simulink model "Detumble_HIL"  (R2020a)
settings: Solver=ode4  StartTime=0.0  StopTime=10  FixedStep=0.05  RelTol=1e-3
values from neighbouring files (symbols this model uses):
  E_b_ECI = [phi_b_ECI; theta_b_ECI; psi_b_ECI]    [Detumble_Initial.m]
  epsilon_b_ECI = [(C_b_ECI(2,3)-C_b_ECI(3,2))/(4*eta_b_ECI) ... (first row only)    [Detumble_Initial.m]
  eta_b_ECI = ((trace(C_b_ECI) + 1)^0.5)/2    [Detumble_Initial.m]
  omega_b_ECI = [-0.05; 0.03; 0.2]    [Detumble_Initial.m]
  state0 = [omega_b_ECI; E_b_ECI; epsilon_b_ECI; eta_b_ECI]    [Detumble_Initial.m]
undefined symbols (not defined in the file or in its folder): Com2, DiscIntNeverNeededParam, none
libraries: xpcseriallib x5
settings Model: SimulationMode=external  Creator=sheab  LastModifiedBy=sheab
settings SolverCC: ConcurrentTasks=on  AutoInsertRateTranBlk=on
settings DataIOCC: SaveFormat=StructureWithTime  SaveOutput=off
settings OptimizationCC: BlockReduction=off  OptimizeBlockIOStorage=off
settings HardwareCC: ProdBitPerPointer=32  ProdBitPerSizeT=32  ProdBitPerPtrDiffT=32  ProdLargestAtomicFloat=None  ProdWordSize=32  ProdLongLongMode=on  ProdHWDeviceType=Generic->32-bit x86 compatible
settings RTWCC: Description=Simulink Real-Time  SystemTargetFile=slrt.tlc  TemplateMakefile=slrt_default_tmf  CodeExecutionProfiling=on  RTWCompilerOptimization=on
settings SimulinkRealTimeCC: SupportVariableSizeSignals=on  RL32LogTETModifier=off  xPCConcurrentTasks=on

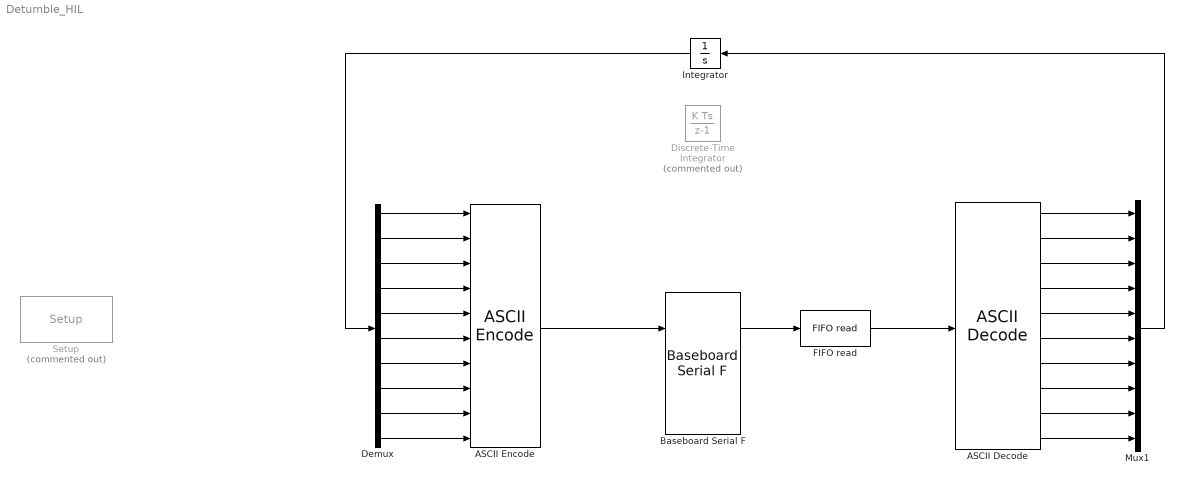
== system Detumble_HIL ==
  "ASCII Decode " : xpcseriallib/ASCII Decode   format=%f %f %f %f %f %f %f %f %f %f\n  nvars=10  vartypes={}
      settings: SourceProductBaseCode=XP
  "ASCII Encode " : xpcseriallib/ASCII Encode   format=%f %f %f %f %f %f %f %f %f %f \n  nvars=10  maxlength=128  vartypes={ 'double' }
      settings: SourceProductBaseCode=XP
  Baseboard Serial F : xpcseriallib/Mainboard/Baseboard Serial F  group=FIFO Setup  port=1  irqnum=4  saddr1=0x3f8  saddr2=0x3e8  config=Com2/none  baud1=115200  parity1=None  ndata1=8  nstop1=1  fifomode1=16 deep  rlevel1=half full  automode1=off  xmtfifosize1=1024  xmtdatatype1=8 bit uint null terminated  rcvfifosize1=5120  baud2=115200  parity2=None  ndata2=8  nstop2=1  fifomode2=16 deep  rlevel2=half full  automode2=off  xmtfifosize2=1024  xmtdatatype2=8 bit uint null terminated  rcvfifosize2=1024
      settings: SourceProductBaseCode=XP
  Demux : Demux  Outputs=10
  Discrete-Time Integrator : DiscreteIntegrator  Commented=on  InitialCondition=[omega_b_ECI; E_b_ECI; epsilon_b_ECI; eta_b_ECI]  SampleTime=-1  SaturateOnIntegerOverflow=on  ICPrevOutput=DiscIntNeverNeededParam  ICPrevScaledInput=DiscIntNeverNeededParam
  "FIFO read " : xpcseriallib/FIFO read   maxsize=5028  minsize=1  usedelimiter=on  delimiter=10  outputtype=8 bit uint null terminated  enable=off  enableout=off  sampletime=0.01
      settings: SourceProductBaseCode=XP
  Integrator : Integrator  Priority=5  InitialCondition=state0
  Mux1 : Mux  Inputs=10
  Setup : xpcseriallib/Mainboard/Baseboard Serial Internal  blocks/Setup  Commented=on  baud=115200  width=8  nstop=1  parity=None  fmode=16 deep  rlevel=half full  ctsmode=on  addr=0x2F8
      settings: SourceProductBaseCode=XP
  wires:
  "ASCII Encode "/1 -> Baseboard Serial F/1
  Baseboard Serial F/1 -> "FIFO read "/1
  Mux1/1 -> Integrator/1
  "ASCII Decode "/10 -> Mux1/10
  "ASCII Decode "/7 -> Mux1/7
  "ASCII Decode "/6 -> Mux1/6
  "ASCII Decode "/9 -> Mux1/9
  "ASCII Decode "/2 -> Mux1/2
  "ASCII Decode "/3 -> Mux1/3
  "ASCII Decode "/1 -> Mux1/1
  "FIFO read "/1 -> "ASCII Decode "/1
  "ASCII Decode "/8 -> Mux1/8
  "ASCII Decode "/4 -> Mux1/4
  "ASCII Decode "/5 -> Mux1/5
  Integrator/1 -> Demux/1
  Demux/5 -> "ASCII Encode "/5
  Demux/4 -> "ASCII Encode "/4
  Demux/2 -> "ASCII Encode "/2
  Demux/3 -> "ASCII Encode "/3
  Demux/1 -> "ASCII Encode "/1
  Demux/6 -> "ASCII Encode "/6
  Demux/7 -> "ASCII Encode "/7
  Demux/8 -> "ASCII Encode "/8
  Demux/9 -> "ASCII Encode "/9
  Demux/10 -> "ASCII Encode "/10
